simulink model "Phase_Recovery_Decision_Directed_Costas_Loop"  (Simulink 8.6)
settings: Solver=FixedStepDiscrete  StartTime=0  StopTime=inf  RelTol=1e-3
InitFcn:
  | % Trainingssequenz
  | trainseq=1/sqrt(2) * ((2*randi([0 1],32,1)-1) + 1i * (2*randi([0 1],32,1)-1));
libraries: commdigbbndpm3 x2, commchan3 x1, dspsrcs4 x1, commsink2 x1, simulink x1, commrandsrc2 x1
settings Model: Creator=schwall  LastModifiedBy=wunsch
settings DataIOCC: SaveOutput=off  SignalLogging=off  SaveTime=off
settings DebuggingCC: InheritedTsInSrcMsg=none  FcnCallInpInsideContextMsg=UseLocalSettings
settings SFSimCC: SimParseCustomCode=off
settings ConfigComp: CovSFcnEnable=off

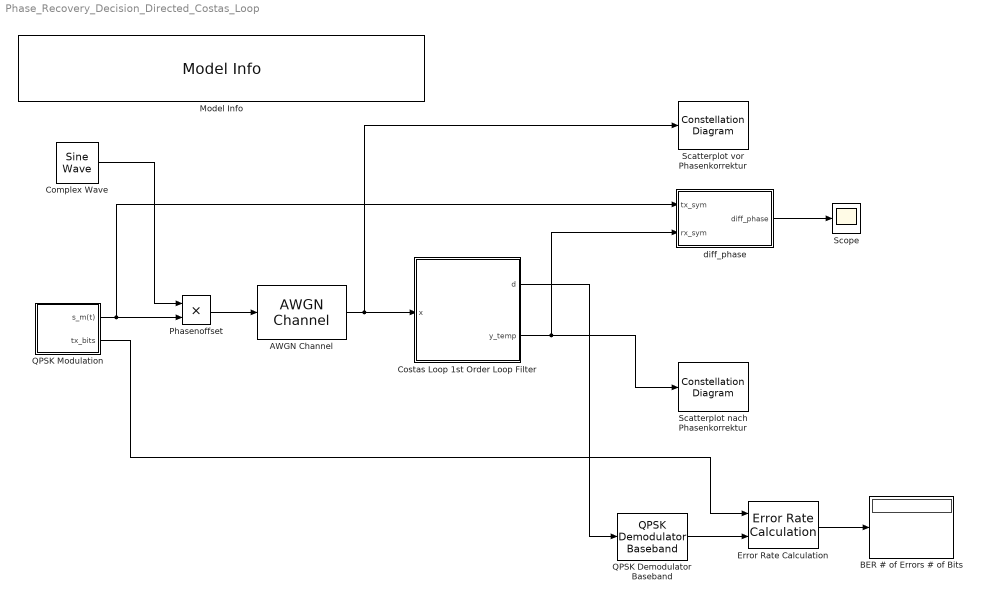
== system Phase_Recovery_Decision_Directed_Costas_Loop ==
  AWGN Channel : commchan3/AWGN Channel  InputProcessing=Columns as channels (frame based)  seed=67  noiseMode="Signal to noise ratio  (Es/No)"  EbNodB=12  EsNodB=20  SNRdB=10  bitsPerSym=2  Ps=1  Tsym=0.128/128  variance=1
  BER # of Errors # of Bits : Display
  Complex Wave : dspsrcs4/Sine Wave  Amplitude=1  Frequency=0  Phase=0  SampleMode=Discrete  OutComplex=Complex  CompMethod=Trigonometric fcn  TableSize=Speed  SampleTime=0.128/128  SamplesPerFrame=128  ResetState=Restart at time zero  OutputFrames=on  dataType=double  wordLen=16  udDataType=sfix(16)  fracBitsMode=Best precision  numFracBits=15  OutDataTypeStr=double  LastOutDataTypeStr=double
  Costas Loop 1st Order Loop Filter : MATLAB Function  TreatAsAtomicUnit=on
  Error Rate Calculation : commsink2/Error Rate Calculation  N=0  st_delay=0  cp_mode=Entire frame  subframe=[]  PMode=Port  WsName=ErrorVec  RsMode2=off  stop=off  numErr=100  maxBits=1e6
  Model Info : simulink/Model-Wide Utilities/Model Info  BlockCM=None  Frame=on  DisplayStringWithTags=|  HorizontalTextAlignment=Left  LeftAlignmentValue=0.02  SourceBlockDiagram=Phase_Recovery_Decision_Directed_Costas_Loop  TagMaxNumber=20
      | Demo Phase Recovery (Costas Loop)
      | Vorlesung Nachrichtentechnik II
      | Institut fuer Nachrichtentechnik (CEL)
  Phasenoffset : Product  RndMeth=Zero
  QPSK Demodulator Baseband : commdigbbndpm3/QPSK Demodulator Baseband  Ph=pi/4  Dec=Gray  OutType=Bit  DecType=Hard decision  VarSource=Dialog  Variance=1  outDtype1=Inherit via internal rule  outDtype2=Inherit via internal rule  derotateFactorWordLen=16
  QPSK Modulation : Subsystem
  Scatterplot nach Phasenkorrektur : ConstellationDiagram  Tag=ScatterPlot
  Scatterplot vor Phasenkorrektur : ConstellationDiagram  Tag=ScatterPlot
  Scope : Scope
  diff_phase : Subsystem
  wires:
  QPSK Modulation/1(s_m(t)) -> Phasenoffset/2, diff_phase/1(tx_sym)
  Costas Loop 1st Order Loop Filter/1(d) -> QPSK Demodulator Baseband/1
  AWGN Channel/1 -> Costas Loop 1st Order Loop Filter/1(x), Scatterplot vor Phasenkorrektur/1
  Phasenoffset/1 -> AWGN Channel/1
  Complex Wave/1 -> Phasenoffset/1
  Costas Loop 1st Order Loop Filter/2(y_temp) -> Scatterplot nach Phasenkorrektur/1, diff_phase/2(rx_sym)
  QPSK Demodulator Baseband/1 -> Error Rate Calculation/2
  QPSK Modulation/2(tx_bits) -> Error Rate Calculation/1
  Error Rate Calculation/1 -> BER # of Errors # of Bits/1
  diff_phase/1(diff_phase) -> Scope/1

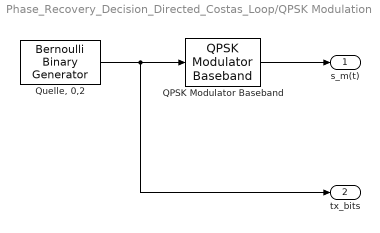
== system Phase_Recovery_Decision_Directed_Costas_Loop/QPSK Modulation ==
  QPSK Modulator Baseband : commdigbbndpm3/QPSK Modulator Baseband  InType=Bit  Enc=Gray  Ph=pi/4  outDtype=double  outWordLen=16  outUDDataType=sfix(16)  outFracLenMode=Best precision  outFracLen=15
  "Quelle, 0,2" : commrandsrc2/Bernoulli Binary Generator  P=0.5  seed=61  Ts=1/1000/2  frameBased=on  sampPerFrame=256  orient=off  outDataType=double
  s_m(t) : Outport
  tx_bits : Outport  Port=2
  wires:
  "Quelle, 0,2"/1 -> QPSK Modulator Baseband/1, tx_bits/1
  QPSK Modulator Baseband/1 -> s_m(t)/1

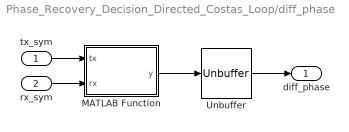
== system Phase_Recovery_Decision_Directed_Costas_Loop/diff_phase ==
  tx_sym : Inport
  rx_sym : Inport  Port=2
  MATLAB Function : MATLAB Function  TreatAsAtomicUnit=on
  Unbuffer : Unbuffer  SampleBasedProcessing=Same as frame based
  diff_phase : Outport
  wires:
  MATLAB Function/1(y) -> Unbuffer/1
  tx_sym/1 -> MATLAB Function/1(tx)
  rx_sym/1 -> MATLAB Function/2(rx)
  Unbuffer/1 -> diff_phase/1

== matlab function diff_phase/MATLAB Function ==
  data: tx input double; y output double; rx input double
function y = fcn(tx,rx)
%#codegen

y=angle(conj(tx).*rx);

== matlab function Costas Loop 1st Order Loop Filter ==
  data: x input double; d output double; y_temp output double
function [d,y_temp] = recovery(x)
%#codegen

%%%%%%%%%%%%%%%%%%%%%%%%%%%%%%%%%%%%%%%%%%%%%%%%%%%%%%%%%%%%%%%%%%%%%%%%%%%
% Initalisierung
%%%%%%%%%%%%%%%%%%%%%%%%%%%%%%%%%%%%%%%%%%%%%%%%%%%%%%%%%%%%%%%%%%%%%%%%%%%

gamma       = 0.1;                          % Schrittweite

persistent phi
if isempty(phi)
    phi = 0;
end

d = complex(zeros(length(x),1));            % Ausgabevektor

y_temp=complex(zeros(length(x),1));         % nur fuer Visualisierungszwecke

%%%%%%%%%%%%%%%%%%%%%%%%%%%%%%%%%%%%%%%%%%%%%%%%%%%%%%%%%%%%%%%%%%%%%%%%%%%
% Phasenkorrektur
%%%%%%%%%%%%%%%%%%%%%%%%%%%%%%%%%%%%%%%%%%%%%%%%%%%%%%%%%%%%%%%%%%%%%%%%%%%

for ii=1:length(x)
    
    
    % Korrektur des Eingangswertes
    y = x(ii) * exp(1i*(-phi));
    
    % nur fuer Visualisierungszwecke
    y_temp(ii) = y;
    
    % Detektor
    d(ii) = detector(y);
    
      
    % Bestimmung des Phasenkorrekturwertes
    phi = phi + gamma * imag( conj(d(ii)) * y );
    
    
end

end


%%%%%%%%%%%%%%%%%%%%%%%%%%%%%%%%%%%%%%%%%%%%%%%%%%%%%%%%%%%%%%%%%%%%%%%%%%%
% QPSK-Detektor
%%%%%%%%%%%%%%%%%%%%%%%%%%%%%%%%%%%%%%%%%%%%%%%%%%%%%%%%%%%%%%%%%%%%%%%%%%%
function d = detector(y)

    % Ueberpruefung der Entscheidungsgebiete
    if     (real(y) >= 0 && imag(y) >= 0)
        d = 1/sqrt(2) * (1+1i);
    elseif (real(y)  < 0 && imag(y) >= 0)
        d = 1/sqrt(2) * (-1+1i);
    elseif (real(y)  < 0 && imag(y)  < 0)
        d = 1/sqrt(2) * (-1-1i);
    else
        d = 1/sqrt(2) * (1-1i);
    end
end
